simulink model "cube0_pd"  (R2019a)
settings: Solver=VariableStepAuto  StartTime=0.0  StopTime=10  RelTol=1e-3  AbsTol=1e-3
undefined symbols (not defined in the file): tar
settings Model: Creator=Abhijit  LastModifiedBy=abhij
settings SolverCC: AutoScaleAbsTol=off
settings DataIOCC: FinalStateName=states  SaveState=on  StateSaveName=states
settings DebuggingCC: SymbolicDimsDataTypeCodeGenerationDiagnostic=none
settings SimscapeCC: SimscapeLogType=all  SimscapeLogSimulationStatistics=on  SimscapeLogDataHistory=10000

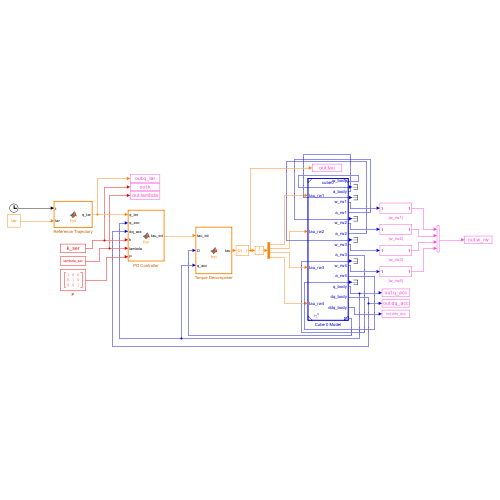
[thumbnail: Simulink's stored preview of the top-level diagram]
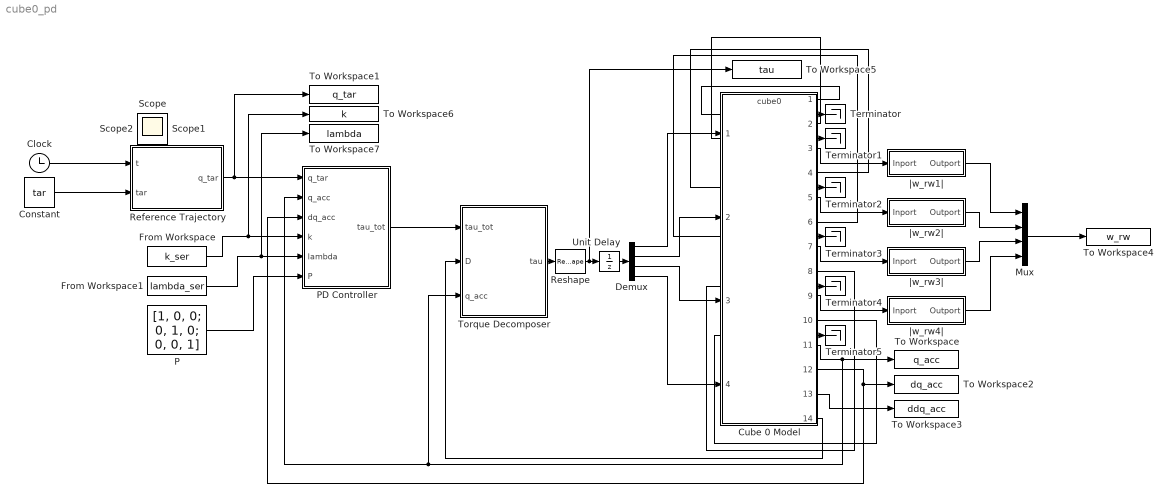
== system cube0_pd ==
  Clock : Clock
  Constant : Constant  Value=tar
  Cube 0 Model : ModelReference  ModelNameDialog=cube0.slx  SimulationMode=Normal  ModelReferenceVersion=1.25
  Demux : Demux
  From Workspace : FromWorkspace  VariableName=k_ser  Interpolate=off  OutputAfterFinalValue=Holding final value
  From Workspace1 : FromWorkspace  VariableName=lambda_ser
  Mux : Mux
  P : Constant  Value=[1, 0, 0; 0, 1, 0; 0, 0, 1]
  PD Controller : MATLAB Function  TreatAsAtomicUnit=on
  Reference Trajectory : MATLAB Function  TreatAsAtomicUnit=on
  Reshape : Reshape
  Terminator{,1..5} (6 alike) : Terminator
  To Workspace : ToWorkspace  VariableName=q_acc  SaveFormat=Timeseries  SampleTime=-1
  To Workspace1 : ToWorkspace  VariableName=q_tar  SaveFormat=Timeseries  SampleTime=-1
  To Workspace2 : ToWorkspace  VariableName=dq_acc  SaveFormat=Timeseries  SampleTime=-1
  To Workspace3 : ToWorkspace  VariableName=ddq_acc  SaveFormat=Timeseries  SampleTime=-1
  To Workspace4 : ToWorkspace  VariableName=w_rw  SaveFormat=Timeseries  SampleTime=-1
  To Workspace5 : ToWorkspace  VariableName=tau  SaveFormat=Timeseries  SampleTime=-1
  To Workspace6 : ToWorkspace  VariableName=k  SaveFormat=Timeseries  SampleTime=-1
  To Workspace7 : ToWorkspace  VariableName=lambda  SaveFormat=Timeseries  SampleTime=-1
  Torque Decomposer : MATLAB Function  TreatAsAtomicUnit=on
  Unit Delay : UnitDelay  SampleTime=-1  HasFrameUpgradeWarning=on
  |w_rw1| : Subsystem
  |w_rw2| : Subsystem
  |w_rw3| : Subsystem
  |w_rw4| : Subsystem
  Scope : Scope
  Scope1 : Scope
  Scope2 : Scope
  wires:
  Cube 0 Model/11 -> To Workspace/1, PD Controller/2(q_acc), Torque Decomposer/3(q_acc)
  |w_rw4|/1(Outport) -> Mux/4
  Cube 0 Model/9 -> |w_rw4|/1(Inport)
  Cube 0 Model/7 -> |w_rw3|/1(Inport)
  Demux/2 -> Cube 0 Model/2
  Reference Trajectory/1(q_tar) -> PD Controller/1(q_tar), To Workspace1/1
  From Workspace/1 -> PD Controller/4(k), To Workspace6/1
  From Workspace1/1 -> To Workspace7/1, PD Controller/5(lambda)
  Mux/1 -> To Workspace4/1
  Demux/4 -> Cube 0 Model/4
  Cube 0 Model/12 -> To Workspace2/1, PD Controller/3(dq_acc)
  Cube 0 Model/14 -> Torque Decomposer/2(D)
  Cube 0 Model/13 -> To Workspace3/1
  Cube 0 Model/5 -> |w_rw2|/1(Inport)
  PD Controller/1(tau_tot) -> Torque Decomposer/1(tau_tot)
  |w_rw2|/1(Outport) -> Mux/2
  |w_rw3|/1(Outport) -> Mux/3
  Clock/1 -> Reference Trajectory/1(t)
  Demux/1 -> Cube 0 Model/1
  Cube 0 Model/3 -> |w_rw1|/1(Inport)
  Demux/3 -> Cube 0 Model/3
  P/1 -> PD Controller/6(P)
  |w_rw1|/1(Outport) -> Mux/1
  Constant/1 -> Reference Trajectory/2(tar)
  Torque Decomposer/1(tau) -> Reshape/1
  Reshape/1 -> Unit Delay/1, To Workspace5/1
  Cube 0 Model/1 -> Terminator/1
  Cube 0 Model/2 -> Terminator1/1
  Cube 0 Model/4 -> Terminator2/1
  Cube 0 Model/6 -> Terminator3/1
  Cube 0 Model/8 -> Terminator4/1
  Cube 0 Model/10 -> Terminator5/1
  Unit Delay/1 -> Demux/1

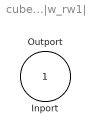
== system cube0_pd/|w_rw1| ==
  Inport : Inport
  Outport : Outport

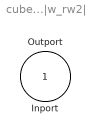
== system cube0_pd/|w_rw2| ==
  Inport : Inport
  Outport : Outport

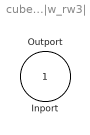
== system cube0_pd/|w_rw3| ==
  Inport : Inport
  Outport : Outport

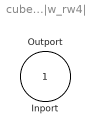
== system cube0_pd/|w_rw4| ==
  Inport : Inport
  Outport : Outport

== matlab function cube0_pd/PD Controller ==
  data: tau_tot output; q_tar input; q_acc input; dq_acc input; k input; lambda input; P input
function tau_tot = fcn(q_tar, q_acc, dq_acc, k, lambda, P)
    tau_tot = pdcontroller(q_tar, q_acc, dq_acc, k, lambda, P);
end

== matlab function cube0_pd/Reference Trajectory ==
  settings: updateMethod=CONTINUOUS
  data: t input; q_tar output; tar input
function q_tar = fcn(t, tar)
     q_tar = refpath(t, tar);
end

== matlab function cube0_pd/Torque Decomposer ==
  data: tau_tot input; tau output; D input; q_acc input
function tau = fcn(tau_tot, D, q_acc)
    tau = taudecomp(tau_tot, D, q_acc);
end
